simulink model "CO2"  (R2018a)
settings: Solver=VariableStepAuto  StartTime=0.0  StopTime=10.0  RelTol=1e-3
settings Model: Creator=e0154145  LastModifiedBy=e0154145

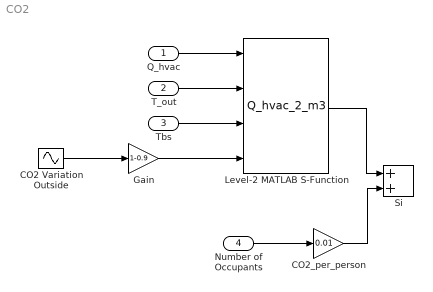
== system CO2 ==
  Q_hvac : Inport
  T_out : Inport  Port=2
  Tbs : Inport  Port=3
  Number of Occupants : Inport  Port=4
  CO2 Variation Outside : Sin  Amplitude=500  Bias=400  Frequency=2*pi/(12*3600)  SampleTime=0
  CO2_per_person : Gain  Gain=0.01
  Gain : Gain  Gain=1-0.9
  Level-2 MATLAB S-Function : M-S-Function  FunctionName=Q_hvac_2_m3
  Si : Sum
  wires:
  Q_hvac/1 -> Level-2 MATLAB S-Function/1
  T_out/1 -> Level-2 MATLAB S-Function/2
  Tbs/1 -> Level-2 MATLAB S-Function/3
  CO2 Variation Outside/1 -> Gain/1
  Level-2 MATLAB S-Function/1 -> Si/1
  Gain/1 -> Level-2 MATLAB S-Function/4
  Number of Occupants/1 -> CO2_per_person/1
  CO2_per_person/1 -> Si/2
